simulink model "DB_1"  (R2018a)
settings: Solver=VariableStepAuto  StartTime=0.0  StopTime=10.0  RelTol=1e-3
values from neighbouring files (symbols this model uses):
  b = 1.1    [Problema1.m]    (also in Problema2.m)
  J = 15    [Problema1.m]    (also in Problema2.m)
  k = 6.8    [Problema1.m]    (also in Problema2.m = 20)
  L = 2.96e-3    (= 0.00296)    [Problema1.m]    (also in Problema2.m)
  R = 0.0435    [Problema1.m]    (also in Problema2.m)
settings Model: Creator=valen  LastModifiedBy=valen
settings DataIOCC: Refine=3

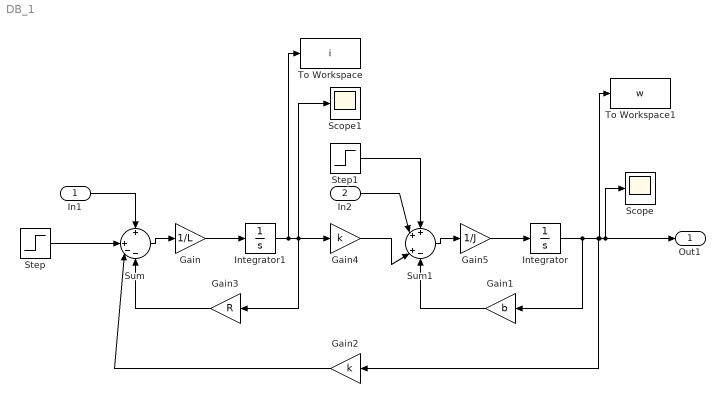
== system DB_1 ==
  In1 : Inport
  In2 : Inport  Port=2
  Gain : Gain  Gain=1/L
  Gain1 : Gain  Gain=b
  Gain2 : Gain  Gain=k
  Gain3 : Gain  Gain=R
  Gain4 : Gain  Gain=k
  Gain5 : Gain  Gain=1/J
  Integrator : Integrator  InitialCondition=65
  Integrator1 : Integrator  InitialCondition=10
  Scope : Scope
  Scope1 : Scope
  Step : Step  Time=0.1  After=0  SampleTime=0
  Step1 : Step  Time=0.1  After=0  SampleTime=0
  Sum : Sum  Inputs=+|+--
  Sum1 : Sum  Inputs=++|+-
  To Workspace : ToWorkspace  VariableName=i  SampleTime=-1
  To Workspace1 : ToWorkspace  VariableName=w  SampleTime=-1
  Out1 : Outport
  wires:
  Sum1/1 -> Gain5/1
  Sum/1 -> Gain/1
  Gain/1 -> Integrator1/1
  Integrator1/1 -> To Workspace/1, Scope1/1, Gain3/1, Gain4/1
  Gain5/1 -> Integrator/1
  Integrator/1 -> Gain1/1, Gain2/1, To Workspace1/1, Scope/1, Out1/1
  In1/1 -> Sum/1
  Gain3/1 -> Sum/4
  Gain2/1 -> Sum/3
  Step/1 -> Sum/2
  Gain1/1 -> Sum1/4
  Gain4/1 -> Sum1/3
  In2/1 -> Sum1/2
  Step1/1 -> Sum1/1
